simulink model "EnergyMonitor_ThreePhase_20s"  (R2022b)
settings: Solver=ode23  StartTime=0.0  StopTime=20.0  MaxStep=1e-3  RelTol=1e-3
settings Model: Creator=User  LastModifiedBy=User

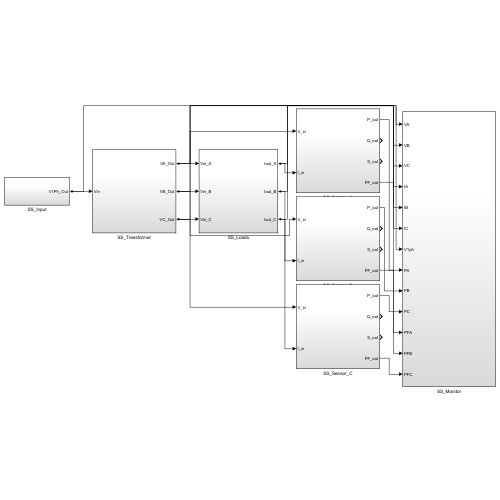
[thumbnail: Simulink's stored preview of the top-level diagram]
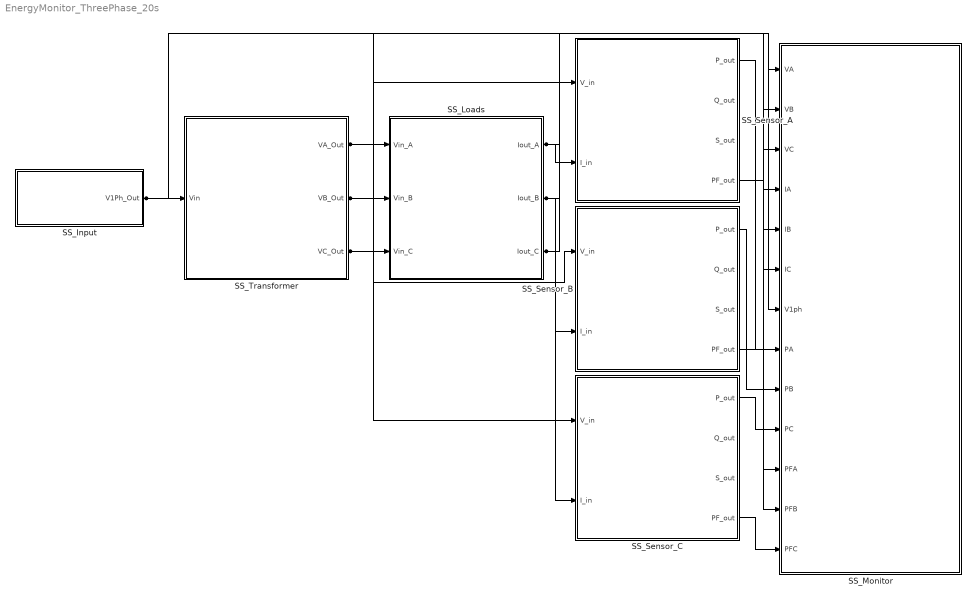
== system EnergyMonitor_ThreePhase_20s ==
  SS_Input : Subsystem
  SS_Loads : Subsystem
  SS_Monitor : Subsystem
  SS_Sensor_A : Subsystem
  SS_Sensor_B : Subsystem
  SS_Sensor_C : Subsystem
  SS_Transformer : Subsystem
  wires:
  SS_Input/1(V1Ph_Out) -> SS_Transformer/1(Vin), SS_Monitor/7(V1ph)
  SS_Transformer/1(VA_Out) -> SS_Loads/1(Vin_A), SS_Monitor/1(VA), SS_Sensor_A/1(V_in)
  SS_Transformer/2(VB_Out) -> SS_Loads/2(Vin_B), SS_Monitor/2(VB), SS_Sensor_B/1(V_in)
  SS_Transformer/3(VC_Out) -> SS_Loads/3(Vin_C), SS_Monitor/3(VC), SS_Sensor_C/1(V_in)
  SS_Loads/1(Iout_A) -> SS_Monitor/4(IA), SS_Sensor_A/2(I_in)
  SS_Loads/2(Iout_B) -> SS_Monitor/5(IB), SS_Sensor_B/2(I_in)
  SS_Loads/3(Iout_C) -> SS_Monitor/6(IC), SS_Sensor_C/2(I_in)
  SS_Sensor_A/1(P_out) -> SS_Monitor/8(PA)
  SS_Sensor_B/1(P_out) -> SS_Monitor/9(PB)
  SS_Sensor_C/1(P_out) -> SS_Monitor/10(PC)
  SS_Sensor_A/4(PF_out) -> SS_Monitor/11(PFA)
  SS_Sensor_B/4(PF_out) -> SS_Monitor/12(PFB)
  SS_Sensor_C/4(PF_out) -> SS_Monitor/13(PFC)

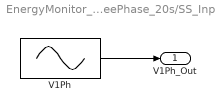
== system EnergyMonitor_ThreePhase_20s/SS_Input ==
  V1Ph : Sin  Amplitude=325.269119  Frequency=314.159265  SampleTime=0
  V1Ph_Out : Outport
  wires:
  V1Ph/1 -> V1Ph_Out/1

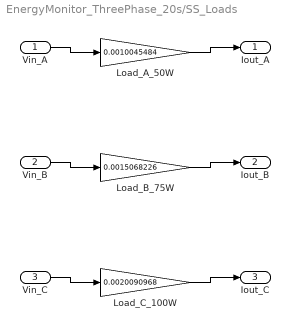
== system EnergyMonitor_ThreePhase_20s/SS_Loads ==
  Vin_A : Inport
  Vin_B : Inport  Port=2
  Vin_C : Inport  Port=3
  Load_A_50W : Gain  Gain=0.0010045484
  Load_B_75W : Gain  Gain=0.0015068226
  Load_C_100W : Gain  Gain=0.0020090968
  Iout_A : Outport
  Iout_B : Outport  Port=2
  Iout_C : Outport  Port=3
  wires:
  Vin_A/1 -> Load_A_50W/1
  Load_A_50W/1 -> Iout_A/1
  Vin_B/1 -> Load_B_75W/1
  Load_B_75W/1 -> Iout_B/1
  Vin_C/1 -> Load_C_100W/1
  Load_C_100W/1 -> Iout_C/1

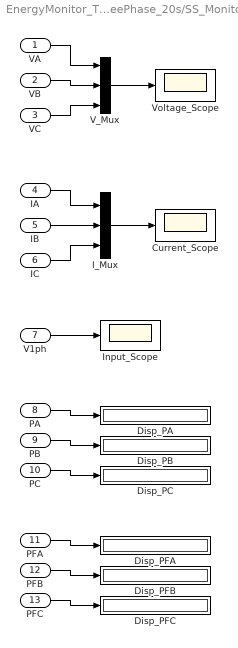
== system EnergyMonitor_ThreePhase_20s/SS_Monitor ==
  VA : Inport
  VB : Inport  Port=2
  VC : Inport  Port=3
  IA : Inport  Port=4
  IB : Inport  Port=5
  IC : Inport  Port=6
  V1ph : Inport  Port=7
  PA : Inport  Port=8
  PB : Inport  Port=9
  PC : Inport  Port=10
  PFA : Inport  Port=11
  PFB : Inport  Port=12
  PFC : Inport  Port=13
  Current_Scope : Scope
  Disp_PA : Display
  Disp_PB : Display
  Disp_PC : Display
  Disp_PFA : Display
  Disp_PFB : Display
  Disp_PFC : Display
  I_Mux : Mux  Inputs=3
  Input_Scope : Scope
  V_Mux : Mux  Inputs=3
  Voltage_Scope : Scope
  wires:
  VA/1 -> V_Mux/1
  VB/1 -> V_Mux/2
  VC/1 -> V_Mux/3
  V_Mux/1 -> Voltage_Scope/1
  IA/1 -> I_Mux/1
  IB/1 -> I_Mux/2
  IC/1 -> I_Mux/3
  I_Mux/1 -> Current_Scope/1
  V1ph/1 -> Input_Scope/1
  PA/1 -> Disp_PA/1
  PB/1 -> Disp_PB/1
  PC/1 -> Disp_PC/1
  PFA/1 -> Disp_PFA/1
  PFB/1 -> Disp_PFB/1
  PFC/1 -> Disp_PFC/1

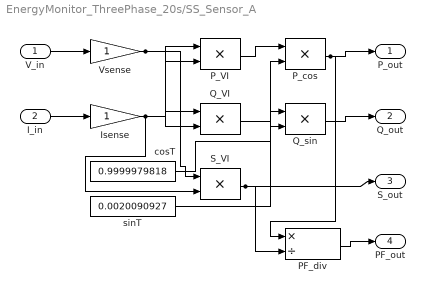
== system EnergyMonitor_ThreePhase_20s/SS_Sensor_A ==
  V_in : Inport
  I_in : Inport  Port=2
  Isense : Gain
  PF_div : Product  Inputs=*/
  P_VI : Product  Inputs=**
  P_cos : Product  Inputs=**
  Q_VI : Product  Inputs=**
  Q_sin : Product  Inputs=**
  S_VI : Product  Inputs=**
  Vsense : Gain
  cosT : Constant  Value=0.9999979818
  sinT : Constant  Value=0.0020090927
  P_out : Outport
  Q_out : Outport  Port=2
  S_out : Outport  Port=3
  PF_out : Outport  Port=4
  wires:
  V_in/1 -> Vsense/1
  I_in/1 -> Isense/1
  Vsense/1 -> P_VI/1, Q_VI/1, S_VI/1
  Isense/1 -> P_VI/2, Q_VI/2, S_VI/2
  P_VI/1 -> P_cos/1
  cosT/1 -> P_cos/2
  P_cos/1 -> P_out/1, PF_div/1
  Q_VI/1 -> Q_sin/1
  sinT/1 -> Q_sin/2
  Q_sin/1 -> Q_out/1
  S_VI/1 -> S_out/1, PF_div/2
  PF_div/1 -> PF_out/1

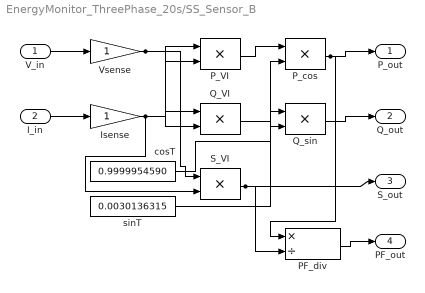
== system EnergyMonitor_ThreePhase_20s/SS_Sensor_B ==
  V_in : Inport
  I_in : Inport  Port=2
  Isense : Gain
  PF_div : Product  Inputs=*/
  P_VI : Product  Inputs=**
  P_cos : Product  Inputs=**
  Q_VI : Product  Inputs=**
  Q_sin : Product  Inputs=**
  S_VI : Product  Inputs=**
  Vsense : Gain
  cosT : Constant  Value=0.9999954590
  sinT : Constant  Value=0.0030136315
  P_out : Outport
  Q_out : Outport  Port=2
  S_out : Outport  Port=3
  PF_out : Outport  Port=4
  wires:
  V_in/1 -> Vsense/1
  I_in/1 -> Isense/1
  Vsense/1 -> P_VI/1, Q_VI/1, S_VI/1
  Isense/1 -> P_VI/2, Q_VI/2, S_VI/2
  P_VI/1 -> P_cos/1
  cosT/1 -> P_cos/2
  P_cos/1 -> P_out/1, PF_div/1
  Q_VI/1 -> Q_sin/1
  sinT/1 -> Q_sin/2
  Q_sin/1 -> Q_out/1
  S_VI/1 -> S_out/1, PF_div/2
  PF_div/1 -> PF_out/1

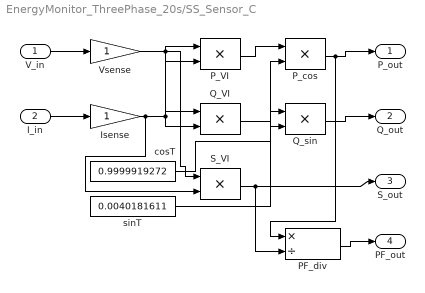
== system EnergyMonitor_ThreePhase_20s/SS_Sensor_C ==
  V_in : Inport
  I_in : Inport  Port=2
  Isense : Gain
  PF_div : Product  Inputs=*/
  P_VI : Product  Inputs=**
  P_cos : Product  Inputs=**
  Q_VI : Product  Inputs=**
  Q_sin : Product  Inputs=**
  S_VI : Product  Inputs=**
  Vsense : Gain
  cosT : Constant  Value=0.9999919272
  sinT : Constant  Value=0.0040181611
  P_out : Outport
  Q_out : Outport  Port=2
  S_out : Outport  Port=3
  PF_out : Outport  Port=4
  wires:
  V_in/1 -> Vsense/1
  I_in/1 -> Isense/1
  Vsense/1 -> P_VI/1, Q_VI/1, S_VI/1
  Isense/1 -> P_VI/2, Q_VI/2, S_VI/2
  P_VI/1 -> P_cos/1
  cosT/1 -> P_cos/2
  P_cos/1 -> P_out/1, PF_div/1
  Q_VI/1 -> Q_sin/1
  sinT/1 -> Q_sin/2
  Q_sin/1 -> Q_out/1
  S_VI/1 -> S_out/1, PF_div/2
  PF_div/1 -> PF_out/1

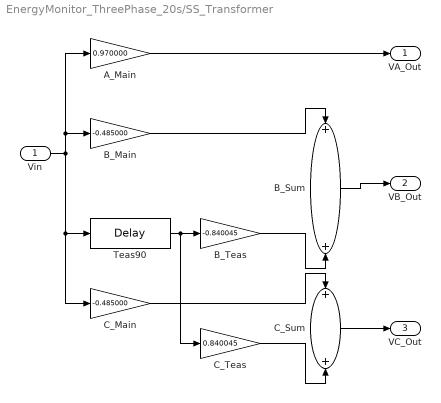
== system EnergyMonitor_ThreePhase_20s/SS_Transformer ==
  Vin : Inport
  A_Main : Gain  Gain=0.970000
  B_Main : Gain  Gain=-0.485000
  B_Sum : Sum
  B_Teas : Gain  Gain=-0.840045
  C_Main : Gain  Gain=-0.485000
  C_Sum : Sum
  C_Teas : Gain  Gain=0.840045
  Teas90 : TransportDelay  DelayTime=0.00500000
  VA_Out : Outport
  VB_Out : Outport  Port=2
  VC_Out : Outport  Port=3
  wires:
  Vin/1 -> Teas90/1, C_Main/1, A_Main/1, B_Main/1
  Teas90/1 -> B_Teas/1, C_Teas/1
  B_Main/1 -> B_Sum/1
  B_Teas/1 -> B_Sum/2
  C_Main/1 -> C_Sum/1
  C_Teas/1 -> C_Sum/2
  A_Main/1 -> VA_Out/1
  B_Sum/1 -> VB_Out/1
  C_Sum/1 -> VC_Out/1
